simulink model "DAS"  (R2012b)
settings: Solver=FixedStepDiscrete  StartTime=0.0  StopTime=inf  FixedStep=0.1  RelTol=1e-3
PreLoadFcn:
  | if exist('tl_preloadfcn','file'), tl_preloadfcn(gcs,101); end
PostLoadFcn:
  | if exist('tl_postloadfcn','file'), tl_postloadfcn(gcs,101); end
InitFcn:
  | if exist('tlds_init','file'), tlds_init(gcs); end
StartFcn:
  | if exist('tlds_start','file'), tlds_start(gcs); end
StopFcn:
  | if exist('tlds_stop','file'), tlds_stop(gcs); end
undefined symbols (not defined in the file): A, B, C, Dd, DEMO_FAS_Accusti_Threshold_Time, DEMO_FAS_BrakeBooster_Threshold, DEMO_FAS_CC_DELTA, DEMO_FAS_CC_Lvl2_Round, DEMO_FAS_CC_Min_Value, DEMO_FAS_Distance_Treshold_Far, DEMO_FAS_Distance_Treshold_Med, DEMO_FAS_Distance_Treshold_Near, DEMO_FAS_Distronic, DEMO_FAS_Emerg_Brake_Force1, DEMO_FAS_Emerg_Brake_Force2, DEMO_FAS_Emerg_Brake_Time1, DEMO_FAS_Emerg_Brake_Time2, DEMO_FAS_EmergencyBrake, DEMO_FAS_FollowToStop, DEMO_FAS_Limiter, DEMO_FAS_Limiter_DELTA, DEMO_FAS_Neg_Max_ms, DEMO_FAS_Opti_Threshold_Time, DEMO_FAS_Repeater, DEMO_FAS_Repeater_Time, DEMO_FAS_Signdetection, DEMO_FAS_Tempomat
(part 10 of 11)

== system DAS/DEMO_FAS/DEMO_FAS/Subsystem/DEMO_FAS/DEMO_FAS_Funktion/Tempomat/Tempomat_Function/CC_SetValue/CC_ChangeSetValue/CC_ChangeSetValue_Lvl2_Repeater/CountDown_RE ==
  E : Inport
  R : Inport  Port=2
  IV : Inport  Port=3
  LogOp_C : Logic  Description=|  AllPortsSameDT=off  mask(TL_LogicalOperator){data={'logdata',{'plotchannels',[]},'date',734383.73486887733}}
      | Logical operator block of dSPACE TargetLink.
      | 
      | The Logical Operator block performs any of these logical operations on its inputs: AND, OR, NAND, NOR, XOR, and NOT. A nonzero input is treated as TRUE (1), a zero input as FALSE (0). The output depends on the selected operator. The output is 1 if TRUE and 0 if FALSE.
      settings: DeleteFcn=if exist('delete_tlblock','file')==2,delete_tlblock(gcbh);end  NameChangeFcn=if exist('rename_tlblock','file')==2,rename_tlblock(gcbh);end  OpenFcn=if exist('tl_open_blockdlg','file')==2,tl_open_blockdlg(gcbh);else,open_system(gcbh,'parameter');end
      mask Help: eval(['if exist(''tl_online_help'',''file'') == 2, tl_online_help(''Topic'',''TL_LogicalOperator''),else, web([''jar:file:///'',matlabroot,''/help/toolbox/simulink/help.jar!/slref/' lower(get_param(gcbh,'Blocktype')) '.html''], ''-helpbrowser''),end'])
      mask Display: plot([-0.05, 1.05, NaN, -0.05, 1.05],[.01, .01, NaN, .99, .99])
  Memory_C : UnitDelay  Description=|  SampleTime=dT  mask(TL_UnitDelay){data={'logdata',{'plotchannels',[]},'date',734383.73486851854}}
      | Unit Delay block of dSPACE TargetLink.
      | 
      | Output signal is equal to the input signal of the last sample step:
      | 
      |         y(k) = u(k-1).
      | 
      | In the 1st sampling step, the output signal is initialized with 'initial condition':
      | 
      |         y(0) = initial condition
      settings: CopyFcn=if exist('tl_reset_reviewflag') == 2, tl_reset_reviewflag(gcbh); end  DeleteFcn=if exist('delete_tlblock','file')==2,delete_tlblock(gcbh);end  NameChangeFcn=if exist('rename_tlblock','file')==2,rename_tlblock(gcbh);end  OpenFcn=if exist('tl_open_blockdlg','file')==2,tl_open_blockdlg(gcbh);else,open_system(gcbh,'parameter');end
      mask Help: eval(['if exist(''tl_online_help'',''file'') == 2, tl_online_help(''Topic'',''TL_UnitDelay''),else, web([''jar:file:///'',matlabroot,''/help/toolbox/simulink/help.jar!/slref/' lower(get_param(gcbh,'Blocktype')) '.html''], ''-helpbrowser''),end'])
      mask Display: plot([-0.05, 1.05, NaN, -0.05, 1.05],[.01, .01, NaN, .99, .99])
  One_C : Constant  Description=|  mask(TL_Constant){data={'date',734383.73486761574}}
      | Constant block of dSPACE TargetLink.
      | 
      | Output signal keeps the given constant value.
      settings: DeleteFcn=if exist('delete_tlblock','file')==2,delete_tlblock(gcbh);end  NameChangeFcn=if exist('rename_tlblock','file')==2,rename_tlblock(gcbh);end  OpenFcn=if exist('tl_open_blockdlg','file')==2,tl_open_blockdlg(gcbh);else,open_system(gcbh,'parameter');end
      mask Help: eval(['if exist(''tl_online_help'',''file'') == 2, tl_online_help(''Topic'',''TL_Constant''),else, web([''jar:file:///'',matlabroot,''/help/toolbox/simulink/help.jar!/slref/' lower(get_param(gcbh,'Blocktype')) '.html''], ''-helpbrowser''),end'])
      mask Display: plot([-0.05, 1.05, NaN, -0.05, 1.05],[.01, .01, NaN, .99, .99])
  RelOp_C : RelationalOperator  Description=|  Operator=>  mask(TL_RelationalOperator){data={'logdata',{'plotchannels',[]},'date',734383.73486724542}}
      | Relational operator block of dSPACE TargetLink.
      | 
      | This block performs a relational operation on its two inputs u1 and u2 and produces output according to the following table.
      | If the result is TRUE, the output is 1; if FALSE, it is 0.
      | 
      | Operator   Output
      |  ==        TRUE if u1 is equal to u2
      |  !=        TRUE if u1 is not equal to u2
      |  <         TRUE if u1 is less than u2
      |  <=        TRUE if u1 is less than or equal to u2
      |  >=        TRUE if u1 is greater than or equal to u2
      |  >         TRUE if u1 is greater than u2
      settings: DeleteFcn=if exist('delete_tlblock','file')==2,delete_tlblock(gcbh);end  NameChangeFcn=if exist('rename_tlblock','file')==2,rename_tlblock(gcbh);end  OpenFcn=if exist('tl_open_blockdlg','file')==2,tl_open_blockdlg(gcbh);else,open_system(gcbh,'parameter');end
      mask Help: eval(['if exist(''tl_online_help'',''file'') == 2, tl_online_help(''Topic'',''TL_RelationalOperator''),else, web([''jar:file:///'',matlabroot,''/help/toolbox/simulink/help.jar!/slref/' lower(get_param(gcbh,'Blocktype')) '.html''], ''-helpbrowser''),end'])
      mask Display: plot([-0.05, 1.05, NaN, -0.05, 1.05],[.01, .01, NaN, .99, .99])
  RelOp_Y : RelationalOperator  Description=|  Operator=>  mask(TL_RelationalOperator){data={'logdata',{'plotchannels',[]},'date',734383.73387511575}}
      | Relational operator block of dSPACE TargetLink.
      | 
      | This block performs a relational operation on its two inputs u1 and u2 and produces output according to the following table.
      | If the result is TRUE, the output is 1; if FALSE, it is 0.
      | 
      | Operator   Output
      |  ==        TRUE if u1 is equal to u2
      |  !=        TRUE if u1 is not equal to u2
      |  <         TRUE if u1 is less than u2
      |  <=        TRUE if u1 is less than or equal to u2
      |  >=        TRUE if u1 is greater than or equal to u2
      |  >         TRUE if u1 is greater than u2
      settings: DeleteFcn=if exist('delete_tlblock','file')==2,delete_tlblock(gcbh);end  NameChangeFcn=if exist('rename_tlblock','file')==2,rename_tlblock(gcbh);end  OpenFcn=if exist('tl_open_blockdlg','file')==2,tl_open_blockdlg(gcbh);else,open_system(gcbh,'parameter');end
      mask Help: eval(['if exist(''tl_online_help'',''file'') == 2, tl_online_help(''Topic'',''TL_RelationalOperator''),else, web([''jar:file:///'',matlabroot,''/help/toolbox/simulink/help.jar!/slref/' lower(get_param(gcbh,'Blocktype')) '.html''], ''-helpbrowser''),end'])
      mask Display: plot([-0.05, 1.05, NaN, -0.05, 1.05],[.01, .01, NaN, .99, .99])
  Sum_C : Sum  Description=|  Inputs=+-  mask(TL_Sum){data={'logdata',{'plotchannels',[]},'date',734383.73387457174}}
      | Sum block of dSPACE TargetLink.
      | 
      | Output signal is equal to the sum of the input signals.
      | The list of signs is specified according to conventions for Simulink Sum blocks.
      settings: CopyFcn=if exist('tl_reset_reviewflag') == 2, tl_reset_reviewflag(gcbh); end  DeleteFcn=if exist('delete_tlblock','file')==2,delete_tlblock(gcbh);end  NameChangeFcn=if exist('rename_tlblock','file')==2,rename_tlblock(gcbh);end  OpenFcn=if exist('tl_open_blockdlg','file')==2,tl_open_blockdlg(gcbh);else,open_system(gcbh,'parameter');end
      mask Help: eval(['if exist(''tl_online_help'',''file'') == 2, tl_online_help(''Topic'',''TL_Sum''),else, web([''jar:file:///'',matlabroot,''/help/toolbox/simulink/help.jar!/slref/' lower(get_param(gcbh,'Blocktype')) '.html''], ''-helpbrowser''),end'])
      mask Display: plot([-0.05, 1.05, NaN, -0.05, 1.05],[.01, .01, NaN, .99, .99])
  Switch_C : Switch  Description=|  Threshold=1  mask(TL_Switch){data={'logdata',{'plotchannels',[]},'date',734383.73387402773}}
      | Switch block of dSPACE TargetLink.
      | 
      | Passes through input 1 if input 2 is greater than or equal to threshold, otherwise, passes through input 3:
      | 
      | if u2 >= threshold
      |    y = u1;
      | else
      |    y = u3;
      | end
      settings: CopyFcn=if exist('tl_reset_reviewflag') == 2, tl_reset_reviewflag(gcbh); end  DeleteFcn=if exist('delete_tlblock','file')==2,delete_tlblock(gcbh);end  NameChangeFcn=if exist('rename_tlblock','file')==2,rename_tlblock(gcbh);end  OpenFcn=if exist('tl_open_blockdlg','file')==2,tl_open_blockdlg(gcbh);else,open_system(gcbh,'parameter');end
      mask Help: eval(['if exist(''tl_online_help'',''file'') == 2, tl_online_help(''Topic'',''TL_Switch''),else, web([''jar:file:///'',matlabroot,''/help/toolbox/simulink/help.jar!/slref/' lower(get_param(gcbh,'Blocktype')) '.html''], ''-helpbrowser''),end'])
      mask Display: plot([-0.05, 1.05, NaN, -0.05, 1.05],[.01, .01, NaN, .99, .99])
  Switch_R : Switch  Description=|  Threshold=1  mask(TL_Switch){data={'logdata',{'plotchannels',[]},'date',734383.73387312505}}
      | Switch block of dSPACE TargetLink.
      | 
      | Passes through input 1 if input 2 is greater than or equal to threshold, otherwise, passes through input 3:
      | 
      | if u2 >= threshold
      |    y = u1;
      | else
      |    y = u3;
      | end
      settings: CopyFcn=if exist('tl_reset_reviewflag') == 2, tl_reset_reviewflag(gcbh); end  DeleteFcn=if exist('delete_tlblock','file')==2,delete_tlblock(gcbh);end  NameChangeFcn=if exist('rename_tlblock','file')==2,rename_tlblock(gcbh);end  OpenFcn=if exist('tl_open_blockdlg','file')==2,tl_open_blockdlg(gcbh);else,open_system(gcbh,'parameter');end
      mask Help: eval(['if exist(''tl_online_help'',''file'') == 2, tl_online_help(''Topic'',''TL_Switch''),else, web([''jar:file:///'',matlabroot,''/help/toolbox/simulink/help.jar!/slref/' lower(get_param(gcbh,'Blocktype')) '.html''], ''-helpbrowser''),end'])
      mask Display: plot([-0.05, 1.05, NaN, -0.05, 1.05],[.01, .01, NaN, .99, .99])
  Zero_C : Constant  Description=|  Value=0  mask(TL_Constant){data={'date',734383.73387240747}}
      | Constant block of dSPACE TargetLink.
      | 
      | Output signal keeps the given constant value.
      settings: DeleteFcn=if exist('delete_tlblock','file')==2,delete_tlblock(gcbh);end  NameChangeFcn=if exist('rename_tlblock','file')==2,rename_tlblock(gcbh);end  OpenFcn=if exist('tl_open_blockdlg','file')==2,tl_open_blockdlg(gcbh);else,open_system(gcbh,'parameter');end
      mask Help: eval(['if exist(''tl_online_help'',''file'') == 2, tl_online_help(''Topic'',''TL_Constant''),else, web([''jar:file:///'',matlabroot,''/help/toolbox/simulink/help.jar!/slref/' lower(get_param(gcbh,'Blocktype')) '.html''], ''-helpbrowser''),end'])
      mask Display: plot([-0.05, 1.05, NaN, -0.05, 1.05],[.01, .01, NaN, .99, .99])
  Zero_Y : Constant  Tag=COPIED_DURING_UPGRADE  Description=|  Value=eps*100000  mask(TL_Constant){data={'date',734383.73381362273}}
      | Constant block of dSPACE TargetLink.
      | 
      | Output signal keeps the given constant value.
      settings: DeleteFcn=if exist('delete_tlblock','file')==2,delete_tlblock(gcbh);end  NameChangeFcn=if exist('rename_tlblock','file')==2,rename_tlblock(gcbh);end  OpenFcn=if exist('tl_open_blockdlg','file')==2,tl_open_blockdlg(gcbh);else,open_system(gcbh,'parameter');end
      mask Help: eval(['if exist(''tl_online_help'',''file'') == 2, tl_online_help(''Topic'',''TL_Constant''),else, web([''jar:file:///'',matlabroot,''/help/toolbox/simulink/help.jar!/slref/' lower(get_param(gcbh,'Blocktype')) '.html''], ''-helpbrowser''),end'])
      mask Display: plot([-0.05, 1.05, NaN, -0.05, 1.05],[.01, .01, NaN, .99, .99])
  y : Outport  InitialOutput=0
  wires:
  Memory_C/1 -> Switch_C/3, Sum_C/1, RelOp_C/1
  Sum_C/1 -> Switch_C/1
  One_C/1 -> Sum_C/2
  LogOp_C/1 -> Switch_C/2
  Switch_C/1 -> Switch_R/3
  R/1 -> Switch_R/2
  Zero_C/1 -> RelOp_C/2
  Switch_R/1 -> RelOp_Y/1, Memory_C/1
  RelOp_C/1 -> LogOp_C/2
  E/1 -> LogOp_C/1
  IV/1 -> Switch_R/1
  Zero_Y/1 -> RelOp_Y/2
  RelOp_Y/1 -> y/1

== system DAS/DEMO_FAS/DEMO_FAS/Subsystem/DEMO_FAS/DEMO_FAS_Funktion/Tempomat/Tempomat_Function/CC_SetValue/CC_ChangeSetValue/CC_ChangeSetValue_Lvl2_Repeater/SysInit ==
  Memory_Init : UnitDelay  Description=|  InitialCondition=1  SampleTime=dT  mask(TL_UnitDelay){data={'logdata',{'plotchannels',[]},'output',{'type','Bool'},'state',{'type','Bool'},'date',734383.73415}}
      | Unit Delay block of dSPACE TargetLink.
      | 
      | Output signal is equal to the input signal of the last sample step:
      | 
      |         y(k) = u(k-1).
      | 
      | In the 1st sampling step, the output signal is initialized with 'initial condition':
      | 
      |         y(0) = initial condition
      settings: CopyFcn=if exist('tl_reset_reviewflag') == 2, tl_reset_reviewflag(gcbh); end  DeleteFcn=if exist('delete_tlblock','file')==2,delete_tlblock(gcbh);end  NameChangeFcn=if exist('rename_tlblock','file')==2,rename_tlblock(gcbh);end  OpenFcn=if exist('tl_open_blockdlg','file')==2,tl_open_blockdlg(gcbh);else,open_system(gcbh,'parameter');end
      mask Help: eval(['if exist(''tl_online_help'',''file'') == 2, tl_online_help(''Topic'',''TL_UnitDelay''),else, web([''jar:file:///'',matlabroot,''/help/toolbox/simulink/help.jar!/slref/' lower(get_param(gcbh,'Blocktype')) '.html''], ''-helpbrowser''),end'])
      mask Display: plot([-0.05, 1.05, NaN, -0.05, 1.05],[.01, .01, NaN, .99, .99])
  Zero_Init : Constant  Description=|  Value=0  SampleTime=dT  mask(TL_Constant){data={'date',734383.73414928245}}
      | Constant block of dSPACE TargetLink.
      | 
      | Output signal keeps the given constant value.
      settings: DeleteFcn=if exist('delete_tlblock','file')==2,delete_tlblock(gcbh);end  NameChangeFcn=if exist('rename_tlblock','file')==2,rename_tlblock(gcbh);end  OpenFcn=if exist('tl_open_blockdlg','file')==2,tl_open_blockdlg(gcbh);else,open_system(gcbh,'parameter');end
      mask Help: eval(['if exist(''tl_online_help'',''file'') == 2, tl_online_help(''Topic'',''TL_Constant''),else, web([''jar:file:///'',matlabroot,''/help/toolbox/simulink/help.jar!/slref/' lower(get_param(gcbh,'Blocktype')) '.html''], ''-helpbrowser''),end'])
      mask Display: plot([-0.05, 1.05, NaN, -0.05, 1.05],[.01, .01, NaN, .99, .99])
  y : Outport
  wires:
  Zero_Init/1 -> Memory_Init/1
  Memory_Init/1 -> y/1

== system DAS/DEMO_FAS/DEMO_FAS/Subsystem/DEMO_FAS/DEMO_FAS_Funktion/Tempomat/Tempomat_Function/CC_SetValue/CC_ChangeSetValue/CC_ChangeSetValue_Lvl2_Repeater/VERSION_INFO ==
  Copyright : Subsystem
      mask help: Copyright
      mask Display: disp('All copyrights by DaimlerChrysler');

== system DAS/DEMO_FAS/DEMO_FAS/Subsystem/DEMO_FAS/DEMO_FAS_Funktion/Tempomat/Tempomat_Function/CC_SetValue/CC_ChangeSetValue/CC_ChangeSetValue_Lvl2_Repeater/V_SetValueMinus ==
  V_CCSetValue : Inport
  Trigger : TriggerPort
  Data Store Write : DataStoreWrite  Description=|  DataStoreName=DEMO_FAS_V_CCSetValue  mask(TL_DataStoreWrite){data={'date',735342.52886488428}}
      | Data Store Write block of dSPACE TargetLink.
      | Use this block to specify outputs to global variables within the production code application.
      settings: DeleteFcn=if exist('delete_tlblock','file')==2,delete_tlblock(gcbh);end  NameChangeFcn=if exist('rename_tlblock','file')==2,rename_tlblock(gcbh);end  OpenFcn=if exist('tl_open_blockdlg','file')==2,tl_open_blockdlg(gcbh);else,open_system(gcbh,'parameter');end
      mask Help: eval(['if exist(''tl_online_help'',''file'') == 2, tl_online_help(''Topic'',''TL_DataStoreWrite''),else, web([''jar:file:///'',matlabroot,''/help/toolbox/simulink/help.jar!/slref/' lower(get_param(gcbh,'Blocktype')) '.html''], ''-helpbrowser''),end'])
      mask Display: plot([-0.05, 1.05, NaN, -0.05, 1.05],[.01, .01, NaN, .99, .99])
  Parameter : Constant  Description=|  Value=DEMO_FAS_CC_DELTA  SampleTime=-1  mask(TL_Constant){data={'output',{'variable','DEMO_FAS/p/Components/DEMO_FAS_CC_DELTA'},'date',735335.59218509262}}
      | Constant block of dSPACE TargetLink.
      | 
      | Output signal keeps the given constant value.
      settings: DeleteFcn=if exist('delete_tlblock','file')==2,delete_tlblock(gcbh);end  NameChangeFcn=if exist('rename_tlblock','file')==2,rename_tlblock(gcbh);end  OpenFcn=if exist('tl_open_blockdlg','file')==2,tl_open_blockdlg(gcbh);else,open_system(gcbh,'parameter');end
      mask Help: eval(['if exist(''tl_online_help'',''file'') == 2, tl_online_help(''Topic'',''TL_Constant''),else, web([''jar:file:///'',matlabroot,''/help/toolbox/simulink/help.jar!/slref/' lower(get_param(gcbh,'Blocktype')) '.html''], ''-helpbrowser''),end'])
      mask Display: plot([-0.05, 1.05, NaN, -0.05, 1.05],[.01, .01, NaN, .99, .99])
  Sum : Sum  Description=|  Inputs=+-  mask(TL_Sum){data={'logdata',{'plotchannels',[]},'date',735335.59140800929}}
      | Sum block of dSPACE TargetLink.
      | 
      | Output signal is equal to the sum of the input signals.
      | The list of signs is specified according to conventions for Simulink Sum blocks.
      settings: CopyFcn=if exist('tl_reset_reviewflag') == 2, tl_reset_reviewflag(gcbh); end  DeleteFcn=if exist('delete_tlblock','file')==2,delete_tlblock(gcbh);end  NameChangeFcn=if exist('rename_tlblock','file')==2,rename_tlblock(gcbh);end  OpenFcn=if exist('tl_open_blockdlg','file')==2,tl_open_blockdlg(gcbh);else,open_system(gcbh,'parameter');end
      mask Help: eval(['if exist(''tl_online_help'',''file'') == 2, tl_online_help(''Topic'',''TL_Sum''),else, web([''jar:file:///'',matlabroot,''/help/toolbox/simulink/help.jar!/slref/' lower(get_param(gcbh,'Blocktype')) '.html''], ''-helpbrowser''),end'])
      mask Display: plot([-0.05, 1.05, NaN, -0.05, 1.05],[.01, .01, NaN, .99, .99])
  VERSION_INFO : Subsystem  mask(VERSION_INFO_BLOCK){versinfo_data=struct('modname','DEMO_FAS/DEMO_FAS_Funktion/Tempomat/Tempomat_Function/CC_SetValue/CC_ChangeSetValue/CC_ChangeSetValue_Lvl2_Repeater/V_SetValueMinus','version','1.1.1','date','22-Apr-2013','author','YVEDUHR','modtype',3,'variant',0,'remark',{{'~'}},'copyright',['Daimler AG'],'SGMLdescr','','prefix','','pfx_act',0,'ntselect',3,'asize',0), versinfo_string=Model: DEMO_FAS/DEMO_FAS_Funktion/Tempomat/Tempomat_Function/CC_SetValue/CC_ChangeSetValue/CC_ChangeSetValue_Lvl2_Repeater/V_SetValueMinus\nVersion: 1.1.1\nDate: 22-Apr-2013\nAuthor: YVEDUHR\nModule: INTERNAL\n\nAll copyrights by Daimler AG}
      mask prompts: versinfo_data "Mask Parameter 1"; versinfo_string "Mask Parameter 2"
      mask help:
      | This is a Version Info Subsystem (empty)
      | All version Information is stored in Parameter "versinfo_data" and displayed
      settings: OpenFcn=edit_subsys_info('init')
      mask Display: disp(versinfo_string);
  wires:
  V_CCSetValue/1 -> Sum/1
  Parameter/1 -> Sum/2
  Sum/1 -> Data Store Write/1

== system DAS/DEMO_FAS/DEMO_FAS/Subsystem/DEMO_FAS/DEMO_FAS_Funktion/Tempomat/Tempomat_Function/CC_SetValue/CC_ChangeSetValue/CC_ChangeSetValue_Lvl2_Repeater/V_SetValueMinusLvl2 ==
  V_CCSetValue : Inport
  Trigger : TriggerPort
  Constant1 : Constant  Value=10  mask(TL_Constant){data={'date',735353.46330140042}}
      settings: CopyFcn=if exist('tl_reset_reviewflag') == 2, tl_reset_reviewflag(gcbh); end  DeleteFcn=if exist('delete_tlblock','file')==2,delete_tlblock(gcbh);end  NameChangeFcn=if exist('rename_tlblock','file')==2,rename_tlblock(gcbh);end  OpenFcn=if exist('tl_open_blockdlg','file')==2,tl_open_blockdlg(gcbh);else,open_system(gcbh,'parameter');end
      mask Help: eval(['if exist(''tl_online_help'',''file'') == 2, tl_online_help(''Topic'',''TL_Constant''),else, web([''jar:file:///'',matlabroot,''/help/toolbox/simulink/help.jar!/slref/' lower(get_param(gcbh,'Blocktype')) '.html''], ''-helpbrowser''),end'])
      mask Display: plot([-0.05, 1.05, NaN, -0.05, 1.05],[.01, .01, NaN, .99, .99])
  DEMO_FAS_CC_Lvl2_Round : Constant  Description=|  Value=DEMO_FAS_CC_Lvl2_Round  SampleTime=-1  mask(TL_Constant){data={'output',{'variable','DEMO_FAS/p/Components/DEMO_FAS_CC_Lvl2_Round'},'date',735354.40958804393}}
      | Constant block of dSPACE TargetLink.
      | 
      | Output signal keeps the given constant value.
      settings: DeleteFcn=if exist('delete_tlblock','file')==2,delete_tlblock(gcbh);end  NameChangeFcn=if exist('rename_tlblock','file')==2,rename_tlblock(gcbh);end  OpenFcn=if exist('tl_open_blockdlg','file')==2,tl_open_blockdlg(gcbh);else,open_system(gcbh,'parameter');end
      mask Help: eval(['if exist(''tl_online_help'',''file'') == 2, tl_online_help(''Topic'',''TL_Constant''),else, web([''jar:file:///'',matlabroot,''/help/toolbox/simulink/help.jar!/slref/' lower(get_param(gcbh,'Blocktype')) '.html''], ''-helpbrowser''),end'])
      mask Display: plot([-0.05, 1.05, NaN, -0.05, 1.05],[.01, .01, NaN, .99, .99])
  Data Store Write1 : DataStoreWrite  Description=|  DataStoreName=DEMO_FAS_V_CCSetValue  mask(TL_DataStoreWrite){data={'date',735342.52895834495}}
      | Data Store Write block of dSPACE TargetLink.
      | Use this block to specify outputs to global variables within the production code application.
      settings: DeleteFcn=if exist('delete_tlblock','file')==2,delete_tlblock(gcbh);end  NameChangeFcn=if exist('rename_tlblock','file')==2,rename_tlblock(gcbh);end  OpenFcn=if exist('tl_open_blockdlg','file')==2,tl_open_blockdlg(gcbh);else,open_system(gcbh,'parameter');end
      mask Help: eval(['if exist(''tl_online_help'',''file'') == 2, tl_online_help(''Topic'',''TL_DataStoreWrite''),else, web([''jar:file:///'',matlabroot,''/help/toolbox/simulink/help.jar!/slref/' lower(get_param(gcbh,'Blocktype')) '.html''], ''-helpbrowser''),end'])
      mask Display: plot([-0.05, 1.05, NaN, -0.05, 1.05],[.01, .01, NaN, .99, .99])
  Math Function : Math  Description=|  Operator=mod  SaturateOnIntegerOverflow=on  mask(TL_Math){data={'logdata',{'plotchannels',[]},'date',735350.66772384255}}
      | Math block of dSPACE TargetLink.
      | 
      | The Math block outputs the result of the specified math function applied to the input(s). Note that unlike Simulink's Math block, this block does not support complex signals.
      settings: CopyFcn=if exist('tl_reset_reviewflag') == 2, tl_reset_reviewflag(gcbh); end  DeleteFcn=if exist('delete_tlblock','file')==2,delete_tlblock(gcbh);end  NameChangeFcn=if exist('rename_tlblock','file')==2,rename_tlblock(gcbh);end  OpenFcn=if exist('tl_open_blockdlg','file')==2,tl_open_blockdlg(gcbh);else,open_system(gcbh,'parameter');end
      mask Help: eval(['if exist(''tl_online_help'',''file'') == 2, tl_online_help(''Topic'',''TL_Math''),else, web([''jar:file:///'',matlabroot,''/help/toolbox/simulink/help.jar!/slref/' lower(get_param(gcbh,'Blocktype')) '.html''], ''-helpbrowser''),end'])
      mask Display: plot([-0.05, 1.05, NaN, -0.05, 1.05],[.01, .01, NaN, .99, .99])
  Sum : Sum  Description=|  Inputs=+-  mask(TL_Sum){data={'logdata',{'plotchannels',[]},'date',735353.40996819444}}
      | Sum block of dSPACE TargetLink.
      | 
      | Output signal is equal to the sum of the input signals.
      | The list of signs is specified according to conventions for Simulink Sum blocks.
      settings: CopyFcn=if exist('tl_reset_reviewflag') == 2, tl_reset_reviewflag(gcbh); end  DeleteFcn=if exist('delete_tlblock','file')==2,delete_tlblock(gcbh);end  NameChangeFcn=if exist('rename_tlblock','file')==2,rename_tlblock(gcbh);end  OpenFcn=if exist('tl_open_blockdlg','file')==2,tl_open_blockdlg(gcbh);else,open_system(gcbh,'parameter');end
      mask Help: eval(['if exist(''tl_online_help'',''file'') == 2, tl_online_help(''Topic'',''TL_Sum''),else, web([''jar:file:///'',matlabroot,''/help/toolbox/simulink/help.jar!/slref/' lower(get_param(gcbh,'Blocktype')) '.html''], ''-helpbrowser''),end'])
      mask Display: plot([-0.05, 1.05, NaN, -0.05, 1.05],[.01, .01, NaN, .99, .99])
  Switch1 : Switch  Threshold=DEMO_FAS_CC_Min_Value  mask(TL_Switch){data={'threshold',{'variable','DEMO_FAS/p/Components/DEMO_FAS_CC_Min_Value'},'date',735354.40995275462}}
      settings: CopyFcn=if exist('tl_reset_reviewflag') == 2, tl_reset_reviewflag(gcbh); end  DeleteFcn=if exist('delete_tlblock','file')==2,delete_tlblock(gcbh);end  NameChangeFcn=if exist('rename_tlblock','file')==2,rename_tlblock(gcbh);end  OpenFcn=if exist('tl_open_blockdlg','file')==2,tl_open_blockdlg(gcbh);else,open_system(gcbh,'parameter');end
      mask Help: eval(['if exist(''tl_online_help'',''file'') == 2, tl_online_help(''Topic'',''TL_Switch''),else, web([''jar:file:///'',matlabroot,''/help/toolbox/simulink/help.jar!/slref/' lower(get_param(gcbh,'Blocktype')) '.html''], ''-helpbrowser''),end'])
      mask Display: plot([-0.05, 1.05, NaN, -0.05, 1.05],[.01, .01, NaN, .99, .99])
  Switch3 : Switch  Criteria=u2 ~= 0  Threshold=1  mask(TL_Switch){data={'date',735353.4651815393}}
      settings: CopyFcn=if exist('tl_reset_reviewflag') == 2, tl_reset_reviewflag(gcbh); end  DeleteFcn=if exist('delete_tlblock','file')==2,delete_tlblock(gcbh);end  NameChangeFcn=if exist('rename_tlblock','file')==2,rename_tlblock(gcbh);end  OpenFcn=if exist('tl_open_blockdlg','file')==2,tl_open_blockdlg(gcbh);else,open_system(gcbh,'parameter');end
      mask Help: eval(['if exist(''tl_online_help'',''file'') == 2, tl_online_help(''Topic'',''TL_Switch''),else, web([''jar:file:///'',matlabroot,''/help/toolbox/simulink/help.jar!/slref/' lower(get_param(gcbh,'Blocktype')) '.html''], ''-helpbrowser''),end'])
      mask Display: plot([-0.05, 1.05, NaN, -0.05, 1.05],[.01, .01, NaN, .99, .99])
  VERSION_INFO : Subsystem  mask(VERSION_INFO_BLOCK){versinfo_data=struct('modname','DEMO_FAS/DEMO_FAS_Funktion/Tempomat/Tempomat_Function/CC_SetValue/CC_ChangeSetValue/CC_ChangeSetValue_Lvl2_Repeater/V_SetValueMinusLvl2','version','1.1.1','date','22-Apr-2013','author','YVEDUHR','modtype',3,'variant',0,'remark',{{'~'}},'copyright',['Daimler AG'],'SGMLdescr','','prefix','','pfx_act',0,'ntselect',3,'asize',0), versinfo_string=Model: DEMO_FAS/DEMO_FAS_Funktion/Tempomat/Tempomat_Function/CC_SetValue/CC_ChangeSetValue/CC_ChangeSetValue_Lvl2_Repeater/V_SetValueMinusLvl2\nVersion: 1.1.1\nDate: 22-Apr-2013\nAuthor: YVEDUHR\nModule: INTERNAL\n\nAll copyrights by Daimler AG}
      mask prompts: versinfo_data "Mask Parameter 1"; versinfo_string "Mask Parameter 2"
      mask help:
      | This is a Version Info Subsystem (empty)
      | All version Information is stored in Parameter "versinfo_data" and displayed
      settings: OpenFcn=edit_subsys_info('init')
      mask Display: disp(versinfo_string);
  wires:
  Sum/1 -> Switch1/1, Switch1/2
  V_CCSetValue/1 -> Switch1/3, Sum/1, Math Function/1
  DEMO_FAS_CC_Lvl2_Round/1 -> Math Function/2
  Switch1/1 -> Data Store Write1/1
  Math Function/1 -> Switch3/2, Switch3/1
  Constant1/1 -> Switch3/3
  Switch3/1 -> Sum/2

== system DAS/DEMO_FAS/DEMO_FAS/Subsystem/DEMO_FAS/DEMO_FAS_Funktion/Tempomat/Tempomat_Function/CC_SetValue/CC_ChangeSetValue/CC_ChangeSetValue_Lvl2_Repeater/V_SetValuePlus ==
  V_CCSetValue : Inport
  Trigger : TriggerPort
  Data Store Write : DataStoreWrite  Description=|  DataStoreName=DEMO_FAS_V_CCSetValue  mask(TL_DataStoreWrite){data={'date',735342.52895834495}}
      | Data Store Write block of dSPACE TargetLink.
      | Use this block to specify outputs to global variables within the production code application.
      settings: DeleteFcn=if exist('delete_tlblock','file')==2,delete_tlblock(gcbh);end  NameChangeFcn=if exist('rename_tlblock','file')==2,rename_tlblock(gcbh);end  OpenFcn=if exist('tl_open_blockdlg','file')==2,tl_open_blockdlg(gcbh);else,open_system(gcbh,'parameter');end
      mask Help: eval(['if exist(''tl_online_help'',''file'') == 2, tl_online_help(''Topic'',''TL_DataStoreWrite''),else, web([''jar:file:///'',matlabroot,''/help/toolbox/simulink/help.jar!/slref/' lower(get_param(gcbh,'Blocktype')) '.html''], ''-helpbrowser''),end'])
      mask Display: plot([-0.05, 1.05, NaN, -0.05, 1.05],[.01, .01, NaN, .99, .99])
  Parameter : Constant  Description=|  Value=DEMO_FAS_CC_DELTA  SampleTime=-1  mask(TL_Constant){data={'output',{'variable','DEMO_FAS/p/Components/DEMO_FAS_CC_DELTA'},'date',735339.65149907407}}
      | Constant block of dSPACE TargetLink.
      | 
      | Output signal keeps the given constant value.
      settings: DeleteFcn=if exist('delete_tlblock','file')==2,delete_tlblock(gcbh);end  NameChangeFcn=if exist('rename_tlblock','file')==2,rename_tlblock(gcbh);end  OpenFcn=if exist('tl_open_blockdlg','file')==2,tl_open_blockdlg(gcbh);else,open_system(gcbh,'parameter');end
      mask Help: eval(['if exist(''tl_online_help'',''file'') == 2, tl_online_help(''Topic'',''TL_Constant''),else, web([''jar:file:///'',matlabroot,''/help/toolbox/simulink/help.jar!/slref/' lower(get_param(gcbh,'Blocktype')) '.html''], ''-helpbrowser''),end'])
      mask Display: plot([-0.05, 1.05, NaN, -0.05, 1.05],[.01, .01, NaN, .99, .99])
  Sum : Sum  Description=|  mask(TL_Sum){data={'logdata',{'plotchannels',[]},'date',734383.73388289358}}
      | Sum block of dSPACE TargetLink.
      | 
      | Output signal is equal to the sum of the input signals.
      | The list of signs is specified according to conventions for Simulink Sum blocks.
      settings: CopyFcn=if exist('tl_reset_reviewflag') == 2, tl_reset_reviewflag(gcbh); end  DeleteFcn=if exist('delete_tlblock','file')==2,delete_tlblock(gcbh);end  NameChangeFcn=if exist('rename_tlblock','file')==2,rename_tlblock(gcbh);end  OpenFcn=if exist('tl_open_blockdlg','file')==2,tl_open_blockdlg(gcbh);else,open_system(gcbh,'parameter');end
      mask Help: eval(['if exist(''tl_online_help'',''file'') == 2, tl_online_help(''Topic'',''TL_Sum''),else, web([''jar:file:///'',matlabroot,''/help/toolbox/simulink/help.jar!/slref/' lower(get_param(gcbh,'Blocktype')) '.html''], ''-helpbrowser''),end'])
      mask Display: plot([-0.05, 1.05, NaN, -0.05, 1.05],[.01, .01, NaN, .99, .99])
  VERSION_INFO : Subsystem  mask(VERSION_INFO_BLOCK){versinfo_data=struct('modname','DEMO_FAS/DEMO_FAS_Funktion/Tempomat/Tempomat_Function/CC_SetValue/CC_ChangeSetValue/CC_ChangeSetValue_Lvl2_Repeater/V_SetValuePlus','version','1.1.1','date','22-Apr-2013','author','YVEDUHR','modtype',3,'variant',0,'remark',{{'~'}},'copyright',['Daimler AG'],'SGMLdescr','','prefix','','pfx_act',0,'ntselect',3,'asize',0), versinfo_string=Model: DEMO_FAS/DEMO_FAS_Funktion/Tempomat/Tempomat_Function/CC_SetValue/CC_ChangeSetValue/CC_ChangeSetValue_Lvl2_Repeater/V_SetValuePlus\nVersion: 1.1.1\nDate: 22-Apr-2013\nAuthor: YVEDUHR\nModule: INTERNAL\n\nAll copyrights by Daimler AG}
      mask prompts: versinfo_data "Mask Parameter 1"; versinfo_string "Mask Parameter 2"
      mask help:
      | This is a Version Info Subsystem (empty)
      | All version Information is stored in Parameter "versinfo_data" and displayed
      settings: OpenFcn=edit_subsys_info('init')
      mask Display: disp(versinfo_string);
  wires:
  V_CCSetValue/1 -> Sum/1
  Parameter/1 -> Sum/2
  Sum/1 -> Data Store Write/1

== system DAS/DEMO_FAS/DEMO_FAS/Subsystem/DEMO_FAS/DEMO_FAS_Funktion/Tempomat/Tempomat_Function/CC_SetValue/CC_ChangeSetValue/CC_ChangeSetValue_Lvl2_Repeater/V_SetValuePlusLvl2 ==
  V_CCSetValue : Inport
  Trigger : TriggerPort
  DEMO_FAS_CC_Lvl2_Round : Constant  Description=|  Value=DEMO_FAS_CC_Lvl2_Round  SampleTime=-1  mask(TL_Constant){data={'output',{'variable','DEMO_FAS/p/Components/DEMO_FAS_CC_Lvl2_Round'},'date',735354.41741359956}}
      | Constant block of dSPACE TargetLink.
      | 
      | Output signal keeps the given constant value.
      settings: DeleteFcn=if exist('delete_tlblock','file')==2,delete_tlblock(gcbh);end  NameChangeFcn=if exist('rename_tlblock','file')==2,rename_tlblock(gcbh);end  OpenFcn=if exist('tl_open_blockdlg','file')==2,tl_open_blockdlg(gcbh);else,open_system(gcbh,'parameter');end
      mask Help: eval(['if exist(''tl_online_help'',''file'') == 2, tl_online_help(''Topic'',''TL_Constant''),else, web([''jar:file:///'',matlabroot,''/help/toolbox/simulink/help.jar!/slref/' lower(get_param(gcbh,'Blocktype')) '.html''], ''-helpbrowser''),end'])
      mask Display: plot([-0.05, 1.05, NaN, -0.05, 1.05],[.01, .01, NaN, .99, .99])
  Data Store Write : DataStoreWrite  Description=|  DataStoreName=DEMO_FAS_V_CCSetValue  mask(TL_DataStoreWrite){data={'date',735342.52895834495}}
      | Data Store Write block of dSPACE TargetLink.
      | Use this block to specify outputs to global variables within the production code application.
      settings: DeleteFcn=if exist('delete_tlblock','file')==2,delete_tlblock(gcbh);end  NameChangeFcn=if exist('rename_tlblock','file')==2,rename_tlblock(gcbh);end  OpenFcn=if exist('tl_open_blockdlg','file')==2,tl_open_blockdlg(gcbh);else,open_system(gcbh,'parameter');end
      mask Help: eval(['if exist(''tl_online_help'',''file'') == 2, tl_online_help(''Topic'',''TL_DataStoreWrite''),else, web([''jar:file:///'',matlabroot,''/help/toolbox/simulink/help.jar!/slref/' lower(get_param(gcbh,'Blocktype')) '.html''], ''-helpbrowser''),end'])
      mask Display: plot([-0.05, 1.05, NaN, -0.05, 1.05],[.01, .01, NaN, .99, .99])
  Math Function : Math  Description=|  Operator=mod  SaturateOnIntegerOverflow=on  mask(TL_Math){data={'logdata',{'plotchannels',[]},'date',735350.66772384255}}
      | Math block of dSPACE TargetLink.
      | 
      | The Math block outputs the result of the specified math function applied to the input(s). Note that unlike Simulink's Math block, this block does not support complex signals.
      settings: CopyFcn=if exist('tl_reset_reviewflag') == 2, tl_reset_reviewflag(gcbh); end  DeleteFcn=if exist('delete_tlblock','file')==2,delete_tlblock(gcbh);end  NameChangeFcn=if exist('rename_tlblock','file')==2,rename_tlblock(gcbh);end  OpenFcn=if exist('tl_open_blockdlg','file')==2,tl_open_blockdlg(gcbh);else,open_system(gcbh,'parameter');end
      mask Help: eval(['if exist(''tl_online_help'',''file'') == 2, tl_online_help(''Topic'',''TL_Math''),else, web([''jar:file:///'',matlabroot,''/help/toolbox/simulink/help.jar!/slref/' lower(get_param(gcbh,'Blocktype')) '.html''], ''-helpbrowser''),end'])
      mask Display: plot([-0.05, 1.05, NaN, -0.05, 1.05],[.01, .01, NaN, .99, .99])
  Sum : Sum  Description=|  mask(TL_Sum){data={'logdata',{'plotchannels',[]},'date',734383.73388289358}}
      | Sum block of dSPACE TargetLink.
      | 
      | Output signal is equal to the sum of the input signals.
      | The list of signs is specified according to conventions for Simulink Sum blocks.
      settings: CopyFcn=if exist('tl_reset_reviewflag') == 2, tl_reset_reviewflag(gcbh); end  DeleteFcn=if exist('delete_tlblock','file')==2,delete_tlblock(gcbh);end  NameChangeFcn=if exist('rename_tlblock','file')==2,rename_tlblock(gcbh);end  OpenFcn=if exist('tl_open_blockdlg','file')==2,tl_open_blockdlg(gcbh);else,open_system(gcbh,'parameter');end
      mask Help: eval(['if exist(''tl_online_help'',''file'') == 2, tl_online_help(''Topic'',''TL_Sum''),else, web([''jar:file:///'',matlabroot,''/help/toolbox/simulink/help.jar!/slref/' lower(get_param(gcbh,'Blocktype')) '.html''], ''-helpbrowser''),end'])
      mask Display: plot([-0.05, 1.05, NaN, -0.05, 1.05],[.01, .01, NaN, .99, .99])
  Sum1 : Sum  Description=|  Inputs=-+  mask(TL_Sum){data={'logdata',{'plotchannels',[]},'date',735350.67227957177}}
      | Sum block of dSPACE TargetLink.
      | 
      | Output signal is equal to the sum of the input signals.
      | The list of signs is specified according to conventions for Simulink Sum blocks.
      settings: CopyFcn=if exist('tl_reset_reviewflag') == 2, tl_reset_reviewflag(gcbh); end  DeleteFcn=if exist('delete_tlblock','file')==2,delete_tlblock(gcbh);end  NameChangeFcn=if exist('rename_tlblock','file')==2,rename_tlblock(gcbh);end  OpenFcn=if exist('tl_open_blockdlg','file')==2,tl_open_blockdlg(gcbh);else,open_system(gcbh,'parameter');end
      mask Help: eval(['if exist(''tl_online_help'',''file'') == 2, tl_online_help(''Topic'',''TL_Sum''),else, web([''jar:file:///'',matlabroot,''/help/toolbox/simulink/help.jar!/slref/' lower(get_param(gcbh,'Blocktype')) '.html''], ''-helpbrowser''),end'])
      mask Display: plot([-0.05, 1.05, NaN, -0.05, 1.05],[.01, .01, NaN, .99, .99])
  VERSION_INFO : Subsystem  mask(VERSION_INFO_BLOCK){versinfo_data=struct('modname','DEMO_FAS/DEMO_FAS_Funktion/Tempomat/Tempomat_Function/CC_SetValue/CC_ChangeSetValue/CC_ChangeSetValue_Lvl2_Repeater/V_SetValuePlusLvl2','version','1.1.1','date','22-Apr-2013','author','YVEDUHR','modtype',3,'variant',0,'remark',{{'~'}},'copyright',['Daimler AG'],'SGMLdescr','','prefix','','pfx_act',0,'ntselect',3,'asize',0), versinfo_string=Model: DEMO_FAS/DEMO_FAS_Funktion/Tempomat/Tempomat_Function/CC_SetValue/CC_ChangeSetValue/CC_ChangeSetValue_Lvl2_Repeater/V_SetValuePlusLvl2\nVersion: 1.1.1\nDate: 22-Apr-2013\nAuthor: YVEDUHR\nModule: INTERNAL\n\nAll copyrights by Daimler AG}
      mask prompts: versinfo_data "Mask Parameter 1"; versinfo_string "Mask Parameter 2"
      mask help:
      | This is a Version Info Subsystem (empty)
      | All version Information is stored in Parameter "versinfo_data" and displayed
      settings: OpenFcn=edit_subsys_info('init')
      mask Display: disp(versinfo_string);
  wires:
  Sum/1 -> Data Store Write/1
  V_CCSetValue/1 -> Sum/1, Math Function/1
  DEMO_FAS_CC_Lvl2_Round/1 -> Sum1/2, Math Function/2
  Math Function/1 -> Sum1/1
  Sum1/1 -> Sum/2

== system DAS/DEMO_FAS/DEMO_FAS/Subsystem/DEMO_FAS/DEMO_FAS_Funktion/Tempomat/Tempomat_Function/CC_SetValue/CC_ChangeSetValue/CC_ChangeSetValue_Lvl2_no_Repeater/VERSION_INFO ==
  Copyright : Subsystem
      mask help: Copyright
      mask Display: disp('All copyrights by DaimlerChrysler');

== system DAS/DEMO_FAS/DEMO_FAS/Subsystem/DEMO_FAS/DEMO_FAS_Funktion/Tempomat/Tempomat_Function/CC_SetValue/CC_ChangeSetValue/CC_ChangeSetValue_Lvl2_no_Repeater/V_SetValueMinus ==
  V_CCSetValue : Inport
  Trigger : TriggerPort
  Data Store Write1 : DataStoreWrite  Description=|  DataStoreName=DEMO_FAS_V_CCSetValue  mask(TL_DataStoreWrite){data={'date',735342.52895834495}}
      | Data Store Write block of dSPACE TargetLink.
      | Use this block to specify outputs to global variables within the production code application.
      settings: DeleteFcn=if exist('delete_tlblock','file')==2,delete_tlblock(gcbh);end  NameChangeFcn=if exist('rename_tlblock','file')==2,rename_tlblock(gcbh);end  OpenFcn=if exist('tl_open_blockdlg','file')==2,tl_open_blockdlg(gcbh);else,open_system(gcbh,'parameter');end
      mask Help: eval(['if exist(''tl_online_help'',''file'') == 2, tl_online_help(''Topic'',''TL_DataStoreWrite''),else, web([''jar:file:///'',matlabroot,''/help/toolbox/simulink/help.jar!/slref/' lower(get_param(gcbh,'Blocktype')) '.html''], ''-helpbrowser''),end'])
      mask Display: plot([-0.05, 1.05, NaN, -0.05, 1.05],[.01, .01, NaN, .99, .99])
  Parameter : Constant  Description=|  Value=DEMO_FAS_CC_DELTA  SampleTime=-1  mask(TL_Constant){data={'output',{'variable','DEMO_FAS/p/Components/DEMO_FAS_CC_DELTA'},'date',735335.59218509262}}
      | Constant block of dSPACE TargetLink.
      | 
      | Output signal keeps the given constant value.
      settings: DeleteFcn=if exist('delete_tlblock','file')==2,delete_tlblock(gcbh);end  NameChangeFcn=if exist('rename_tlblock','file')==2,rename_tlblock(gcbh);end  OpenFcn=if exist('tl_open_blockdlg','file')==2,tl_open_blockdlg(gcbh);else,open_system(gcbh,'parameter');end
      mask Help: eval(['if exist(''tl_online_help'',''file'') == 2, tl_online_help(''Topic'',''TL_Constant''),else, web([''jar:file:///'',matlabroot,''/help/toolbox/simulink/help.jar!/slref/' lower(get_param(gcbh,'Blocktype')) '.html''], ''-helpbrowser''),end'])
      mask Display: plot([-0.05, 1.05, NaN, -0.05, 1.05],[.01, .01, NaN, .99, .99])
  Sum : Sum  Description=|  Inputs=+-  mask(TL_Sum){data={'logdata',{'plotchannels',[]},'date',735335.59140800929}}
      | Sum block of dSPACE TargetLink.
      | 
      | Output signal is equal to the sum of the input signals.
      | The list of signs is specified according to conventions for Simulink Sum blocks.
      settings: CopyFcn=if exist('tl_reset_reviewflag') == 2, tl_reset_reviewflag(gcbh); end  DeleteFcn=if exist('delete_tlblock','file')==2,delete_tlblock(gcbh);end  NameChangeFcn=if exist('rename_tlblock','file')==2,rename_tlblock(gcbh);end  OpenFcn=if exist('tl_open_blockdlg','file')==2,tl_open_blockdlg(gcbh);else,open_system(gcbh,'parameter');end
      mask Help: eval(['if exist(''tl_online_help'',''file'') == 2, tl_online_help(''Topic'',''TL_Sum''),else, web([''jar:file:///'',matlabroot,''/help/toolbox/simulink/help.jar!/slref/' lower(get_param(gcbh,'Blocktype')) '.html''], ''-helpbrowser''),end'])
      mask Display: plot([-0.05, 1.05, NaN, -0.05, 1.05],[.01, .01, NaN, .99, .99])
  Switch : Switch  Threshold=DEMO_FAS_CC_Min_Value  mask(TL_Switch){data={'threshold',{'variable','DEMO_FAS/p/Components/DEMO_FAS_CC_Min_Value'},'date',735354.41010562505}}
      settings: CopyFcn=if exist('tl_reset_reviewflag') == 2, tl_reset_reviewflag(gcbh); end  DeleteFcn=if exist('delete_tlblock','file')==2,delete_tlblock(gcbh);end  NameChangeFcn=if exist('rename_tlblock','file')==2,rename_tlblock(gcbh);end  OpenFcn=if exist('tl_open_blockdlg','file')==2,tl_open_blockdlg(gcbh);else,open_system(gcbh,'parameter');end
      mask Help: eval(['if exist(''tl_online_help'',''file'') == 2, tl_online_help(''Topic'',''TL_Switch''),else, web([''jar:file:///'',matlabroot,''/help/toolbox/simulink/help.jar!/slref/' lower(get_param(gcbh,'Blocktype')) '.html''], ''-helpbrowser''),end'])
      mask Display: plot([-0.05, 1.05, NaN, -0.05, 1.05],[.01, .01, NaN, .99, .99])
  VERSION_INFO : Subsystem  mask(VERSION_INFO_BLOCK){versinfo_data=struct('modname','DEMO_FAS/DEMO_FAS_Funktion/Tempomat/Tempomat_Function/CC_SetValue/CC_ChangeSetValue/CC_ChangeSetValue_Lvl2_no_Repeater/V_SetValueMinus','version','1.1.1','date','22-Apr-2013','author','YVEDUHR','modtype',3,'variant',0,'remark',{{'~'}},'copyright',['Daimler AG'],'SGMLdescr','','prefix','','pfx_act',0,'ntselect',3,'asize',0), versinfo_string=Model: DEMO_FAS/DEMO_FAS_Funktion/Tempomat/Tempomat_Function/CC_SetValue/CC_ChangeSetValue/CC_ChangeSetValue_Lvl2_no_Repeater/V_SetValueMinus\nVersion: 1.1.1\nDate: 22-Apr-2013\nAuthor: YVEDUHR\nModule: INTERNAL\n\nAll copyrights by Daimler AG}
      mask prompts: versinfo_data "Mask Parameter 1"; versinfo_string "Mask Parameter 2"
      mask help:
      | This is a Version Info Subsystem (empty)
      | All version Information is stored in Parameter "versinfo_data" and displayed
      settings: OpenFcn=edit_subsys_info('init')
      mask Display: disp(versinfo_string);
  wires:
  Parameter/1 -> Sum/2
  V_CCSetValue/1 -> Switch/3, Sum/1
  Sum/1 -> Switch/1, Switch/2
  Switch/1 -> Data Store Write1/1
